simulink model "InvPendulumESP"  (R2023b)
settings: Solver=FixedStepAuto  StartTime=0.0  StopTime=inf  FixedStep=0.01  RelTol=1e-3
values from neighbouring files (symbols this model uses):
  PWMBias = 35    [LQRJoe.m]    (also in LQRScript.m)
  PWMSat = 255    [LQRJoe.m]    (also in LQRScript.m)
undefined symbols (not defined in the file or in its folder): K
libraries: simulink x2, arduinosensorlib x2, arduinolib x2
settings Model: ExtModeTrigDuration=2  Creator=M  LastModifiedBy=abdob
settings SolverCC: AlgebraicLoopSolver=TrustRegion
settings OptimizationCC: EnhancedBackFolding=on  PassReuseOutputArgsAs=Individual arguments  ZeroExternalMemoryAtStartup=off  ZeroInternalMemoryAtStartup=off  MaxStackSize=64  OptimizeBlockOrder=speed  DifferentSizesBufferReuse=on  OptimizationCustomize=off  EfficientTunableParamExpr=on
settings DebuggingCC: ParameterTunabilityLossMsg=error  UnconnectedInputMsg=warning  UnconnectedOutputMsg=warning  UnconnectedLineMsg=warning
settings HardwareCC: ProdBitPerPointer=32  ProdBitPerSizeT=32  ProdBitPerPtrDiffT=32  ProdLargestAtomicInteger=Long  ProdLargestAtomicFloat=Double  ProdWordSize=32  ProdHWDeviceType=ARM Compatible->ARM Cortex
settings ModelReferenceCC: EnableRefExpFcnMdlSchedulingChecks=on
settings SFSimCC: MATLABDynamicMemAlloc=off
settings RTWCC: Description=Embedded Coder  SystemTargetFile=ert.tlc  HardwareBoard=ESP32-WROOM(Arduino Compatible)  TLCOptions="-aInlineSetEventsForThisBaseRateFcn=TLC_FALSE -aSuppressMultiTaskScheduler=TLC_FALSE  -aRateBasedStepFcn=0"  TemplateMakefile=ert_default_tmf  Toolchain=ESP32  BuildConfiguration=Faster Runs
settings CodeAppCC: ForceParamTrailComments=on  IgnoreCustomStorageClasses=off  OperatorAnnotations=on  SimulinkDataObjDesc=on  SFDataObjDesc=on  InsertBlockDesc=on
settings ERTTargetCC: SupportContinuousTime=on  SupportVariableSizeSignals=on  ExtModeTransport=3  ExtModeStaticAlloc=on  ExtModeAutomaticAllocSize=off  ExtModeStaticAllocSize=65536  ExtModeMexFile=ext_xcp  ExtModeIntrfLevel=Level2 - Open

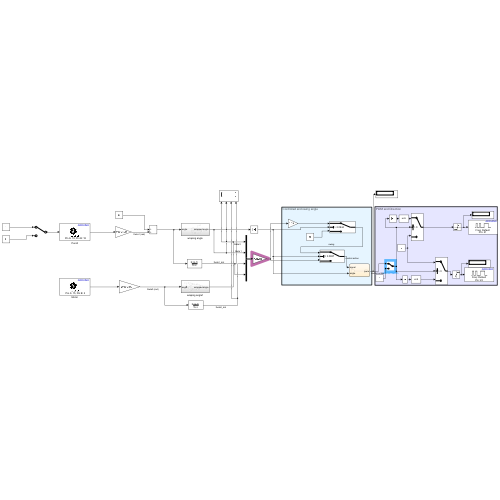
[thumbnail: Simulink's stored preview of the top-level diagram]
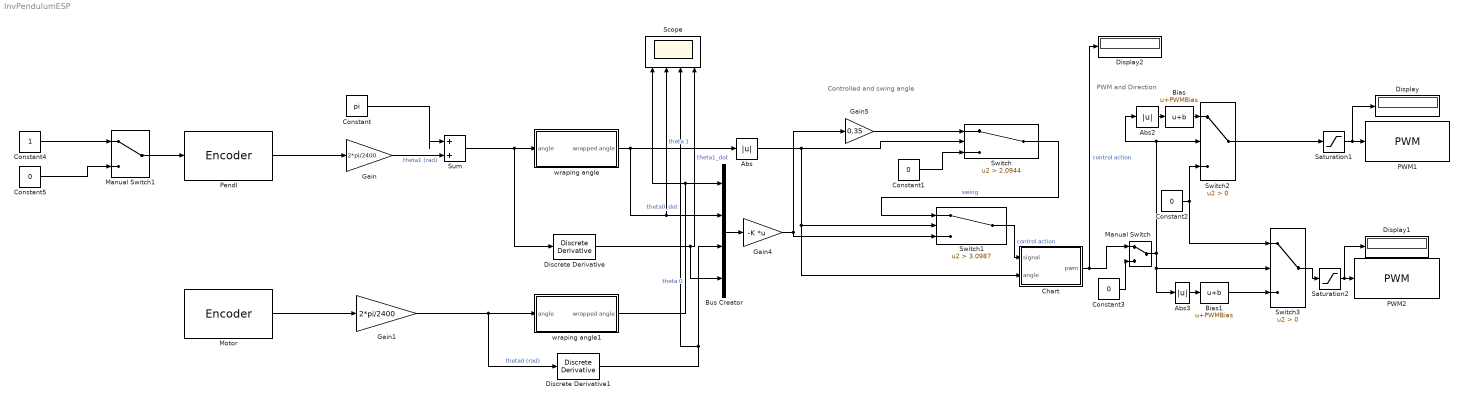
== system InvPendulumESP ==
  note: PWM and Direction
  note: Controlled and swing angle
  Abs : Abs  SaturateOnIntegerOverflow=off
  Abs2 : Abs  SaturateOnIntegerOverflow=off
  Abs3 : Abs  SaturateOnIntegerOverflow=off
  Bias : Bias  Bias=PWMBias  SaturateOnIntegerOverflow=off
  Bias1 : Bias  Bias=PWMBias  SaturateOnIntegerOverflow=off
  Bus Creator : BusCreator  Inputs=4
  Chart : Stateflow chart  TreatAsAtomicUnit=on
  Constant : Constant  Value=pi
  Constant{1..3,5} (4 alike) : Constant  Value=0
  Constant4 : Constant
  Discrete Derivative : simulink/Discrete/Discrete Derivative  gainval=1.0  ICPrevScaledInput=0.0  OutMin=[]  OutMax=[]  OutDataType=fixdt(1, 16)  OutScaling=2^-10  DoSatur=off
  Discrete Derivative1 : simulink/Discrete/Discrete Derivative  gainval=1.0  ICPrevScaledInput=0.0  OutMin=[]  OutMax=[]  OutDataType=fixdt(1, 16)  OutScaling=2^-10  DoSatur=off
  Display : Display
  Display1 : Display
  Display2 : Display
  Gain : Gain  Gain=2*pi/2400  ParamDataTypeStr=double
  Gain1 : Gain  Gain=2*pi/2400  ParamDataTypeStr=double
  Gain4 : Gain  Gain=-K  Multiplication=Matrix(K*u) (u vector)
  Gain5 : Gain  Gain=0.35
  Manual Switch : ManualSwitch
  Manual Switch1 : ManualSwitch
  Motor : arduinosensorlib/Encoder  InputA=15  InputB=2  Mode=No reset  SampleTime=-1
  PWM1 : arduinolib/PWM  pinNumber=21  frequencyType=Default  desiredFrequency=200  achievableFrequency=200
  PWM2 : arduinolib/PWM  pinNumber=22  frequencyType=Default  desiredFrequency=200  achievableFrequency=200
  Pendl : arduinosensorlib/Encoder  InputA=19  InputB=18  Mode=Reset by external signal  SampleTime=-1
  Saturation1 : Saturate  UpperLimit=PWMSat  LowerLimit=0
  Saturation2 : Saturate  UpperLimit=PWMSat  LowerLimit=0
  Scope : Scope  NumInputPorts=4
  Sum : Sum  Inputs=|++
  Switch : Switch  Criteria=u2 > Threshold  Threshold=2.0944  SaturateOnIntegerOverflow=off  InputSameDT=off
  Switch1 : Switch  Criteria=u2 > Threshold  Threshold=3.0987  SaturateOnIntegerOverflow=off  InputSameDT=off
  Switch2 : Switch  Criteria=u2 > Threshold  SaturateOnIntegerOverflow=off  InputSameDT=off
  Switch3 : Switch  Criteria=u2 > Threshold  SaturateOnIntegerOverflow=off  InputSameDT=off
  wraping angle : Subsystem
  wraping angle1 : Subsystem
  wires:
  Motor/1 -> Gain1/1
  Pendl/1 -> Gain/1
  Constant/1 -> Sum/1
  Gain/1 -> Sum/2  "theta1 (rad)"
  Sum/1 -> Discrete Derivative/1, wraping angle/1(angle)
  wraping angle1/1(wrapped angle) -> Bus Creator/1, Scope/1  "theta 0"
  wraping angle/1(wrapped angle) -> Bus Creator/2, Scope/2, Abs/1  "theta 1"
  Gain1/1 -> Discrete Derivative1/1, wraping angle1/1(angle)  "theta0 (rad)"
  Abs/1 -> Chart/2(angle), Switch1/2, Switch/2
  Switch/1 -> Switch1/1  "swing"
  Constant1/1 -> Switch/3
  Gain5/1 -> Switch/1
  Saturation2/1 -> Display1/1, PWM2/1
  Gain4/1 -> Switch1/3, Gain5/1
  Discrete Derivative/1 -> Bus Creator/4, Scope/4  "theta1_dot"
  Discrete Derivative1/1 -> Scope/3, Bus Creator/3  "theta0_dot"
  Constant2/1 -> Switch2/3, Switch3/1
  Saturation1/1 -> Display/1, PWM1/1
  Switch1/1 -> Chart/1(signal)  "control action"
  Bus Creator/1 -> Gain4/1
  Manual Switch/1 -> Abs3/1, Switch3/2, Switch2/2, Abs2/1
  Switch2/1 -> Saturation1/1
  Switch3/1 -> Saturation2/1
  Abs2/1 -> Bias/1
  Bias/1 -> Switch2/1
  Abs3/1 -> Bias1/1
  Bias1/1 -> Switch3/3
  Manual Switch1/1 -> Pendl/1
  Constant5/1 -> Manual Switch1/2
  Constant4/1 -> Manual Switch1/1
  Constant3/1 -> Manual Switch/2
  Chart/1(pwm) -> Display2/1, Manual Switch/1  "control action"

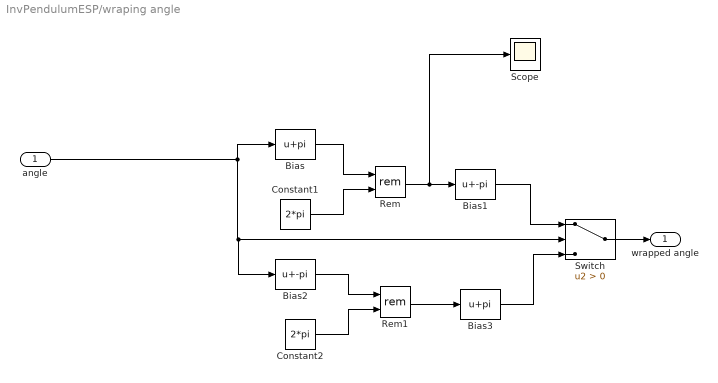
== system InvPendulumESP/wraping angle ==
  angle : Inport
  Bias : Bias  Bias=pi  SaturateOnIntegerOverflow=off
  Bias1 : Bias  Bias=-pi  SaturateOnIntegerOverflow=off
  Bias2 : Bias  Bias=-pi  SaturateOnIntegerOverflow=off
  Bias3 : Bias  Bias=pi  SaturateOnIntegerOverflow=off
  Constant1 : Constant  Value=2*pi
  Constant2 : Constant  Value=2*pi
  Rem : Math  Operator=rem
  Rem1 : Math  Operator=rem
  Scope : Scope
  Switch : Switch  Criteria=u2 > Threshold  SaturateOnIntegerOverflow=off  InputSameDT=off
  wrapped angle : Outport
  wires:
  Bias/1 -> Rem/1
  Rem1/1 -> Bias3/1
  Bias3/1 -> Switch/3
  Constant1/1 -> Rem/2
  Constant2/1 -> Rem1/2
  Bias1/1 -> Switch/1
  Bias2/1 -> Rem1/1
  Rem/1 -> Scope/1, Bias1/1
  Switch/1 -> wrapped angle/1
  angle/1 -> Bias/1, Bias2/1, Switch/2

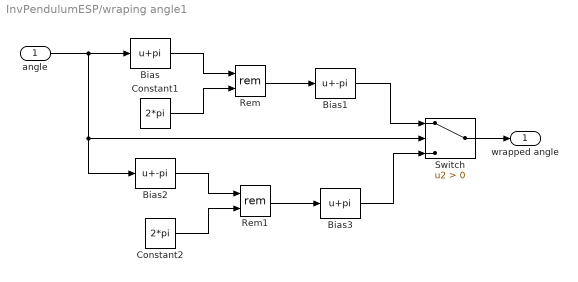
== system InvPendulumESP/wraping angle1 ==
  angle : Inport
  Bias : Bias  Bias=pi  SaturateOnIntegerOverflow=off
  Bias1 : Bias  Bias=-pi  SaturateOnIntegerOverflow=off
  Bias2 : Bias  Bias=-pi  SaturateOnIntegerOverflow=off
  Bias3 : Bias  Bias=pi  SaturateOnIntegerOverflow=off
  Constant1 : Constant  Value=2*pi
  Constant2 : Constant  Value=2*pi
  Rem : Math  Operator=rem
  Rem1 : Math  Operator=rem
  Switch : Switch  Criteria=u2 > Threshold  SaturateOnIntegerOverflow=off  InputSameDT=off
  wrapped angle : Outport
  wires:
  Switch/1 -> wrapped angle/1
  Rem/1 -> Bias1/1
  Bias2/1 -> Rem1/1
  Bias1/1 -> Switch/1
  Constant2/1 -> Rem1/2
  Constant1/1 -> Rem/2
  Bias3/1 -> Switch/3
  Rem1/1 -> Bias3/1
  angle/1 -> Bias/1, Bias2/1, Switch/2
  Bias/1 -> Rem/1

== stateflow chart InvPendulumESP/Chart ==
  note: %%angle < 135
  state start
    pwm = 255
  state stop
    pwm = signal
  (default) -> start
  start -> stop : [angle < (22/7) * (3/4)]
  stop -> start : [[ angle >(22/7)*(3/4)] && after(3,sec)]
  data: signal input; angle input; pwm output
